simulink library "simpleWinch_ul"  (R2018b)
settings: Solver=VariableStepAuto  StartTime=0.0  StopTime=10.0  RelTol=1e-3
settings Model: Creator=Ayaz  LastModifiedBy=Ayaz

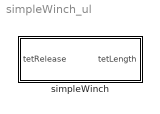
== system simpleWinch_ul ==
  simpleWinch : Subsystem  mask{maxRelease=0, maxTug=0, iniLength=0}
      mask prompts: maxRelease "Winch max release speed"; maxTug "Winch max tug speed"; iniLength "Tether initial length"
      mask init:
      | maxRelease = abs(maxRelease);
      | maxTug = -abs(maxTug);

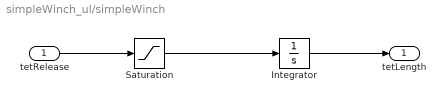
== system simpleWinch_ul/simpleWinch ==
  tetRelease : Inport
  Integrator : Integrator  InitialCondition=iniLength
  Saturation : Saturate  UpperLimit=maxRelease  LowerLimit=maxTug
  tetLength : Outport
  wires:
  tetRelease/1 -> Saturation/1
  Saturation/1 -> Integrator/1
  Integrator/1 -> tetLength/1
